simulink model "Slip_Ratio_Controller"  (R2018b)
settings: Solver=FixedStepAuto  StartTime=0.0  StopTime=10.0  FixedStep=global_time_step  RelTol=1e-3
undefined symbols (not defined in the file): Area, Cd, DiscIntNeverNeededParam, Jw, Mass, Q, r, R, rho, SRC_Ts, tyre_radius
libraries: simulink x2, peGeneralControl x1
settings Model: PauseTimes=1  Creator=univ4123  LastModifiedBy=univ4123
settings RTWCC: GenCodeOnly=on  Toolchain=MinGW64 | gmake (64-bit Windows)

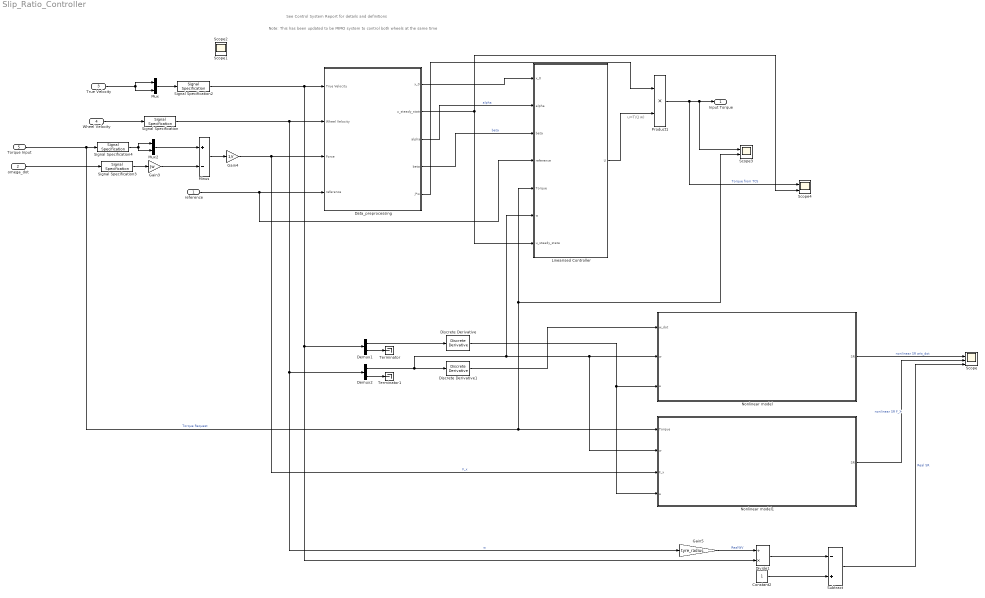
== system Slip_Ratio_Controller ==
  note: Note: This has been updated to be MIMO system to control both wheels at the same time
  note: See Control System Report for details and definitions
  note: u=T/(J w)
  reference : Inport
  omega_dot : Inport  Port=2
  True Velocity : Inport  Port=3
  Wheel Velocity : Inport  Port=4
  Torque Input : Inport  Port=5
  Constant2 : Constant  SampleTime=SRC_Ts
  Data_preprocessing : Subsystem
  Demux1 : Demux  Outputs=2
  Demux2 : Demux  Outputs=2
  Discrete Derivative : simulink/Discrete/Discrete Derivative  gainval=1.0  ICPrevScaledInput=0.0  OutMin=[]  OutMax=[]  OutDataType=fixdt(1, 16)  OutScaling=2^-10  DoSatur=off
  Discrete Derivative1 : simulink/Discrete/Discrete Derivative  gainval=1.0  ICPrevScaledInput=0.0  OutMin=[]  OutMax=[]  OutDataType=fixdt(1, 16)  OutScaling=2^-10  DoSatur=off
  Divide1 : Product  Inputs=/*
  Gain3 : Gain  Gain=Jw
  Gain4 : Gain  Gain=1/r
  Gain5 : Gain  Gain=tyre_radius
  Linearised Controller : Subsystem
  Minus : Sum  Inputs=+-
  Mux : Mux  Inputs=2
  Mux2 : Mux  Inputs=2
  Nonlinear model : Subsystem
  Nonlinear model1 : Subsystem
  Product1 : Product
  Scope : Scope  NumInputPorts=4
  Scope3 : Scope  NumInputPorts=2
  Scope4 : Scope  NumInputPorts=2
  Signal Specification : SignalSpecification  Dimensions=[2,1]
  Signal Specification2 : SignalSpecification  Dimensions=[2,1]
  Signal Specification3 : SignalSpecification  Dimensions=[2,1]
  Signal Specification4 : SignalSpecification  Dimensions=1
  Subtract : Sum  Inputs=-+
  Terminator : Terminator
  Terminator1 : Terminator
  Input Torque : Outport
  Scope1 : Scope
  Scope2 : Scope
  wires:
  Wheel Velocity/1 -> Signal Specification/1
  Data_preprocessing/2(u_steady_state) -> Scope4/2, Linearised Controller/7(u_steady_state)
  Linearised Controller/1(U) -> Product1/2
  Product1/1 -> Scope4/1, Scope3/1, Input Torque/1  "Torque from TCS"
  reference/1 -> Linearised Controller/4(reference), Data_preprocessing/4(reference)
  True Velocity/1 -> Mux/2, Mux/1
  Gain4/1 -> Nonlinear model1/3(F_x), Data_preprocessing/3(Force)  "F_x"
  Nonlinear model/1(SR) -> Scope/2  "nonlinear SR w/w_dot"
  Demux1/2 -> Terminator/1
  Demux2/2 -> Terminator1/1
  Torque Input/1 -> Nonlinear model1/1(Torque), Linearised Controller/5(Torque), Scope3/2, Signal Specification4/1  "Torque Request"
  Demux1/1 -> Discrete Derivative/1
  Demux2/1 -> Nonlinear model1/2(w), Nonlinear model/2(w), Linearised Controller/6(w), Discrete Derivative1/1
  Discrete Derivative/1 -> Nonlinear model1/4(a), Nonlinear model/3(a)
  Discrete Derivative1/1 -> Nonlinear model/1(w_dot)
  Gain3/1 -> Minus/2
  Minus/1 -> Gain4/1
  omega_dot/1 -> Signal Specification3/1
  Mux2/1 -> Minus/1
  Signal Specification3/1 -> Gain3/1
  Signal Specification4/1 -> Mux2/1, Mux2/2
  Nonlinear model1/1(SR) -> Scope/3  "nonlinear SR F_X"
  Signal Specification/1 -> Gain5/1, Demux2/1, Data_preprocessing/2(Wheel Velocity)  "w"
  Divide1/1 -> Subtract/1
  Mux/1 -> Signal Specification2/1
  Gain5/1 -> Divide1/1  "RealWV"
  Constant2/1 -> Subtract/2
  Subtract/1 -> Scope/4  "Real SR"
  Signal Specification2/1 -> Divide1/2, Demux1/1, Data_preprocessing/1(True Velocity)
  Data_preprocessing/1(x_0) -> Linearised Controller/1(x_0)
  Data_preprocessing/3(alpha) -> Linearised Controller/2(alpha)  "alpha"
  Data_preprocessing/4(beta) -> Linearised Controller/3(beta)  "beta"
  Data_preprocessing/5(J*w) -> Product1/1

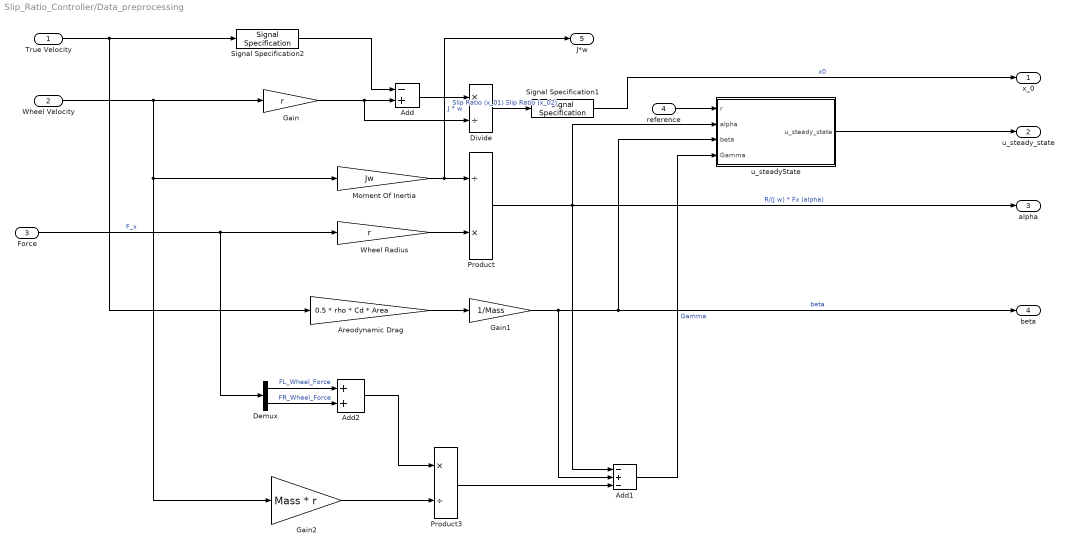
== system Slip_Ratio_Controller/Data_preprocessing ==
  True Velocity : Inport
  Wheel Velocity : Inport  Port=2
  Force : Inport  Port=3
  reference : Inport  Port=4
  Add : Sum  Inputs=-+
  Add1 : Sum  Inputs=-+-
  Add2 : Sum
  Areodynamic Drag : Gain  Gain=0.5 * rho * Cd * Area
  Demux : Demux  Outputs=2
  Divide : Product  Inputs=*/
  Gain : Gain  Gain=r
  Gain1 : Gain  Gain=1/Mass
  Gain2 : Gain  Gain=Mass * r
  Moment Of Inertia : Gain  Gain=Jw
  Product : Product  Inputs=/*
  Product3 : Product  Inputs=*/
  Signal Specification1 : SignalSpecification  Dimensions=[2,1]
  Signal Specification2 : SignalSpecification  Dimensions=[2,1]
  Wheel Radius : Gain  Gain=r
  u_steadyState : Subsystem
  x_0 : Outport
  u_steady_state : Outport  Port=2
  alpha : Outport  Port=3
  beta : Outport  Port=4
  J*w : Outport  Port=5
  wires:
  True Velocity/1 -> Signal Specification2/1, Areodynamic Drag/1
  Signal Specification2/1 -> Add/1
  Wheel Velocity/1 -> Gain/1, Moment Of Inertia/1, Gain2/1
  Product/1 -> u_steadyState/2(alpha), alpha/1, Add1/1  "R/(J w) * Fx (alpha)"
  Moment Of Inertia/1 -> J*w/1, Product/1  "J * w"
  Gain/1 -> Divide/2, Add/2
  Divide/1 -> Signal Specification1/1  "Slip Ratio (x_01) Slip Ratio (x_02)"
  Wheel Radius/1 -> Product/2
  Gain1/1 -> u_steadyState/3(beta), beta/1, Add1/2  "beta"
  Add1/1 -> u_steadyState/4(Gamma)  "Gamma"
  Demux/2 -> Add2/2  "FR_Wheel_Force"
  Add2/1 -> Product3/1
  Gain2/1 -> Product3/2
  Signal Specification1/1 -> x_0/1  "x0"
  Force/1 -> Demux/1, Wheel Radius/1  "F_x"
  Areodynamic Drag/1 -> Gain1/1
  Product3/1 -> Add1/3
  Demux/1 -> Add2/1  "FL_Wheel_Force"
  Add/1 -> Divide/1
  u_steadyState/1(u_steady_state) -> u_steady_state/1
  reference/1 -> u_steadyState/1(r)

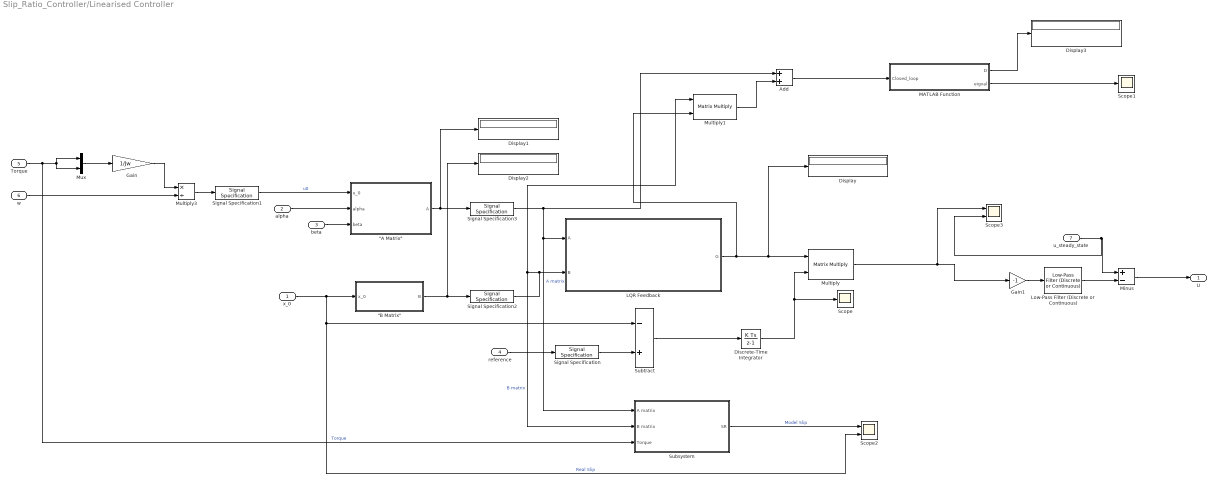
== system Slip_Ratio_Controller/Linearised Controller ==
  x_0 : Inport
  alpha : Inport  Port=2
  beta : Inport  Port=3
  reference : Inport  Port=4
  Torque : Inport  Port=5
  w : Inport  Port=6
  u_steady_state : Inport  Port=7
  "\"A Matrix\"" : Subsystem
  "\"B Matrix\"" : Subsystem
  Add : Sum
  Discrete-Time Integrator : DiscreteIntegrator  SampleTime=-1  ICPrevOutput=DiscIntNeverNeededParam  ICPrevScaledInput=DiscIntNeverNeededParam
  Display{,1..3} (4 alike) : Display
  Gain : Gain  Gain=1/Jw
  Gain1 : Gain  Gain=-1
  LQR Feedback : Subsystem
  Low-Pass Filter (Discrete or Continuous) : peGeneralControl/Low-Pass Filter (Discrete or Continuous)  K=1  T=10  B=inf  A=-inf  Ts=-1
  MATLAB Function : MATLAB Function  TreatAsAtomicUnit=on
  Minus : Sum  Inputs=+-
  Multiply : Product  Multiplication=Matrix(*)
  Multiply1 : Product  Multiplication=Matrix(*)
  Multiply3 : Product  Inputs=*/
  Mux : Mux  Inputs=2
  Scope : Scope
  Scope1 : Scope
  Scope2 : Scope  NumInputPorts=2
  Scope3 : Scope  NumInputPorts=2
  Signal Specification : SignalSpecification  Dimensions=[2 1]
  Signal Specification1 : SignalSpecification  Dimensions=[2,1]
  Signal Specification2 : SignalSpecification  Dimensions=[2,2]
  Signal Specification3 : SignalSpecification  Dimensions=[2,2]
  Subsystem : Subsystem
  Subtract : Sum  Inputs=-+
  U : Outport
  wires:
  alpha/1 -> "\"A Matrix\""/2(alpha)
  beta/1 -> "\"A Matrix\""/3(beta)
  x_0/1 -> Scope2/2, Subtract/1, "\"B Matrix\""/1(x_0)  "Real Slip"
  "\"A Matrix\""/1(A) -> Display1/1, Signal Specification3/1
  "\"B Matrix\""/1(B) -> Display2/1, Signal Specification2/1
  reference/1 -> Signal Specification/1
  Signal Specification2/1 -> LQR Feedback/2(B), Subsystem/2(B matrix), Multiply1/1  "B matrix"
  Signal Specification3/1 -> Add/1, Subsystem/1(A matrix), LQR Feedback/1(A)  "A matrix"
  Multiply3/1 -> Signal Specification1/1
  Gain/1 -> Multiply3/1
  w/1 -> Multiply3/2
  Torque/1 -> Subsystem/3(Torque), Mux/2, Mux/1  "Torque"
  Mux/1 -> Gain/1
  Signal Specification/1 -> Subtract/2
  Signal Specification1/1 -> "\"A Matrix\""/1(u_0)  "u0"
  Low-Pass Filter (Discrete or Continuous)/1 -> Minus/2
  Gain1/1 -> Low-Pass Filter (Discrete or Continuous)/1
  Multiply/1 -> Scope3/1, Gain1/1
  Minus/1 -> U/1
  Subtract/1 -> Discrete-Time Integrator/1
  Discrete-Time Integrator/1 -> Multiply/2, Scope/1
  LQR Feedback/1(G) -> Multiply1/2, Display/1, Multiply/1
  Multiply1/1 -> Add/2
  Add/1 -> MATLAB Function/1(Closed_loop)
  MATLAB Function/1(D) -> Display3/1
  MATLAB Function/2(eigval) -> Scope1/1
  Subsystem/1(SR) -> Scope2/1  "Model Slip"
  u_steady_state/1 -> Scope3/2, Minus/1

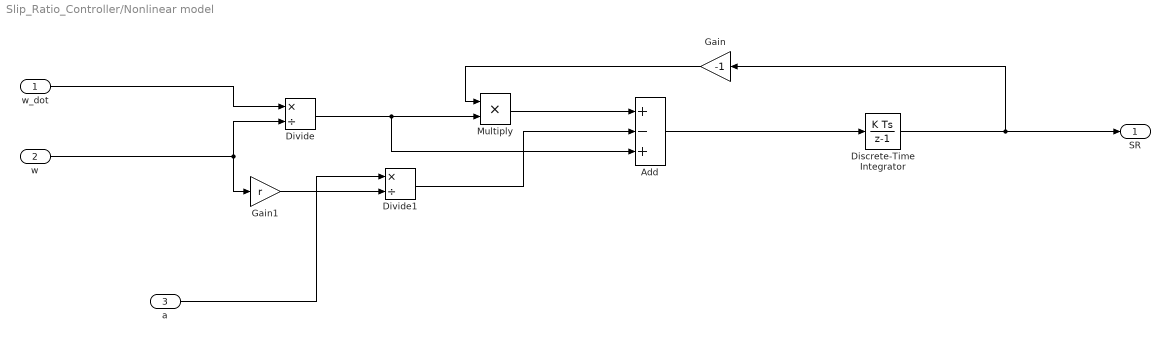
== system Slip_Ratio_Controller/Nonlinear model ==
  w_dot : Inport
  w : Inport  Port=2
  a : Inport  Port=3
  Add : Sum  Inputs=+-+
  Discrete-Time Integrator : DiscreteIntegrator  SampleTime=-1  ICPrevOutput=DiscIntNeverNeededParam  ICPrevScaledInput=DiscIntNeverNeededParam
  Divide : Product  Inputs=*/
  Divide1 : Product  Inputs=*/
  Gain : Gain  Gain=-1
  Gain1 : Gain  Gain=r
  Multiply : Product
  SR : Outport
  wires:
  w_dot/1 -> Divide/1
  w/1 -> Divide/2, Gain1/1
  Gain1/1 -> Divide1/2
  Divide/1 -> Add/3, Multiply/2
  Gain/1 -> Multiply/1
  Multiply/1 -> Add/1
  a/1 -> Divide1/1
  Divide1/1 -> Add/2
  Add/1 -> Discrete-Time Integrator/1
  Discrete-Time Integrator/1 -> Gain/1, SR/1

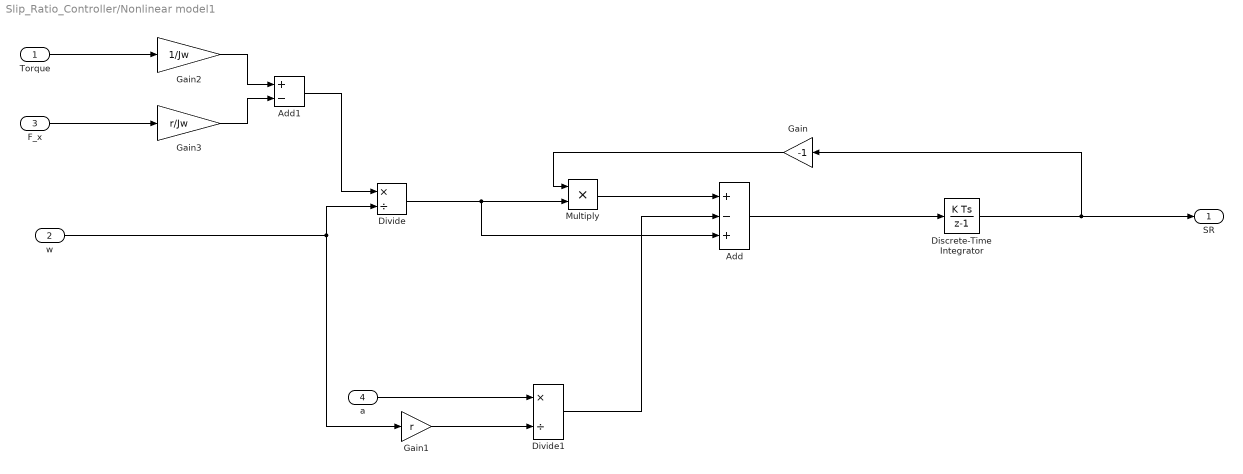
== system Slip_Ratio_Controller/Nonlinear model1 ==
  Torque : Inport
  w : Inport  Port=2
  F_x : Inport  Port=3
  a : Inport  Port=4
  Add : Sum  Inputs=+-+
  Add1 : Sum  Inputs=+-
  Discrete-Time Integrator : DiscreteIntegrator  SampleTime=-1  ICPrevOutput=DiscIntNeverNeededParam  ICPrevScaledInput=DiscIntNeverNeededParam
  Divide : Product  Inputs=*/
  Divide1 : Product  Inputs=*/
  Gain : Gain  Gain=-1
  Gain1 : Gain  Gain=r
  Gain2 : Gain  Gain=1/Jw
  Gain3 : Gain  Gain=r/Jw
  Multiply : Product
  SR : Outport
  wires:
  Torque/1 -> Gain2/1
  w/1 -> Gain1/1, Divide/2
  Gain1/1 -> Divide1/2
  Divide/1 -> Add/3, Multiply/2
  Gain/1 -> Multiply/1
  Multiply/1 -> Add/1
  a/1 -> Divide1/1
  Divide1/1 -> Add/2
  Add/1 -> Discrete-Time Integrator/1
  Discrete-Time Integrator/1 -> Gain/1, SR/1
  F_x/1 -> Gain3/1
  Gain2/1 -> Add1/1
  Gain3/1 -> Add1/2
  Add1/1 -> Divide/1

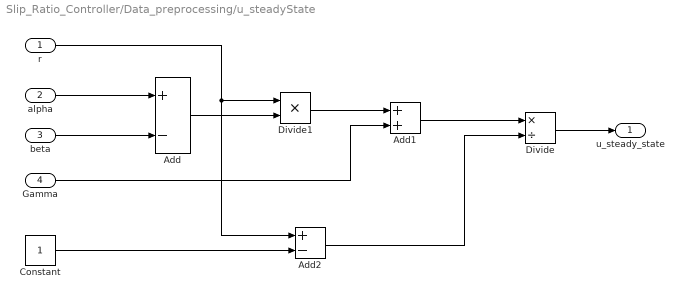
== system Slip_Ratio_Controller/Data_preprocessing/u_steadyState ==
  r : Inport
  alpha : Inport  Port=2
  beta : Inport  Port=3
  Gamma : Inport  Port=4
  Add : Sum  Inputs=+-
  Add1 : Sum
  Add2 : Sum  Inputs=+-
  Constant : Constant  SampleTime=SRC_Ts
  Divide : Product  Inputs=*/
  Divide1 : Product  Inputs=**
  u_steady_state : Outport
  wires:
  Divide/1 -> u_steady_state/1
  Add/1 -> Divide1/2
  alpha/1 -> Add/1
  beta/1 -> Add/2
  r/1 -> Add2/1, Divide1/1
  Divide1/1 -> Add1/1
  Gamma/1 -> Add1/2
  Add1/1 -> Divide/1
  Constant/1 -> Add2/2
  Add2/1 -> Divide/2

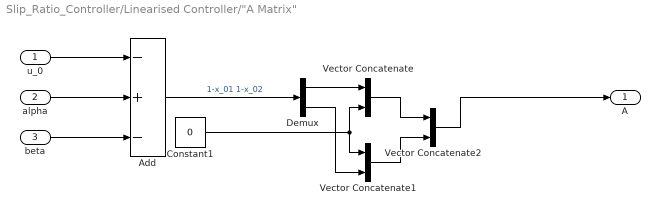
== system Slip_Ratio_Controller/Linearised Controller/"A Matrix" ==
  u_0 : Inport
  alpha : Inport  Port=2
  beta : Inport  Port=3
  Add : Sum  Inputs=-+-
  Constant1 : Constant  Value=0  SampleTime=SRC_Ts
  Demux : Demux  Outputs=2
  Vector Concatenate : Concatenate  ConcatenateDimension=2
  Vector Concatenate1 : Concatenate
  Vector Concatenate2 : Concatenate  Mode=Multidimensional array  ConcatenateDimension=2
  A : Outport
  wires:
  u_0/1 -> Add/1
  alpha/1 -> Add/2
  beta/1 -> Add/3
  Demux/2 -> Vector Concatenate1/2
  Add/1 -> Demux/1  "1-x_01 1-x_02"
  Constant1/1 -> Vector Concatenate1/1, Vector Concatenate/2
  Vector Concatenate1/1 -> Vector Concatenate2/2
  Vector Concatenate2/1 -> A/1
  Demux/1 -> Vector Concatenate/1
  Vector Concatenate/1 -> Vector Concatenate2/1

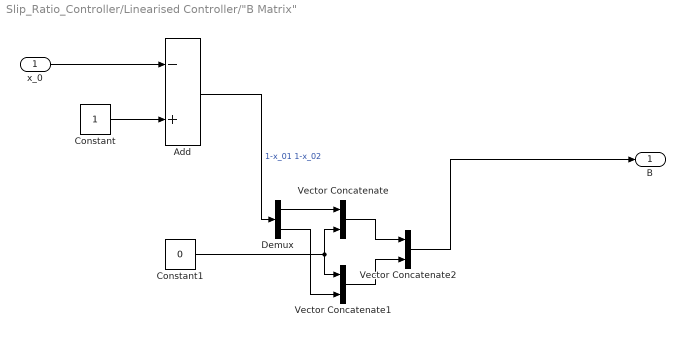
== system Slip_Ratio_Controller/Linearised Controller/"B Matrix" ==
  x_0 : Inport
  Add : Sum  Inputs=-+
  Constant : Constant  SampleTime=SRC_Ts
  Constant1 : Constant  Value=0  SampleTime=SRC_Ts
  Demux : Demux  Outputs=2
  Vector Concatenate : Concatenate  ConcatenateDimension=2
  Vector Concatenate1 : Concatenate
  Vector Concatenate2 : Concatenate  Mode=Multidimensional array  ConcatenateDimension=2
  B : Outport
  wires:
  Constant/1 -> Add/2
  Add/1 -> Demux/1  "1-x_01 1-x_02"
  Demux/1 -> Vector Concatenate/1
  Demux/2 -> Vector Concatenate1/2
  Constant1/1 -> Vector Concatenate1/1, Vector Concatenate/2
  Vector Concatenate1/1 -> Vector Concatenate2/2
  Vector Concatenate/1 -> Vector Concatenate2/1
  Vector Concatenate2/1 -> B/1
  x_0/1 -> Add/1

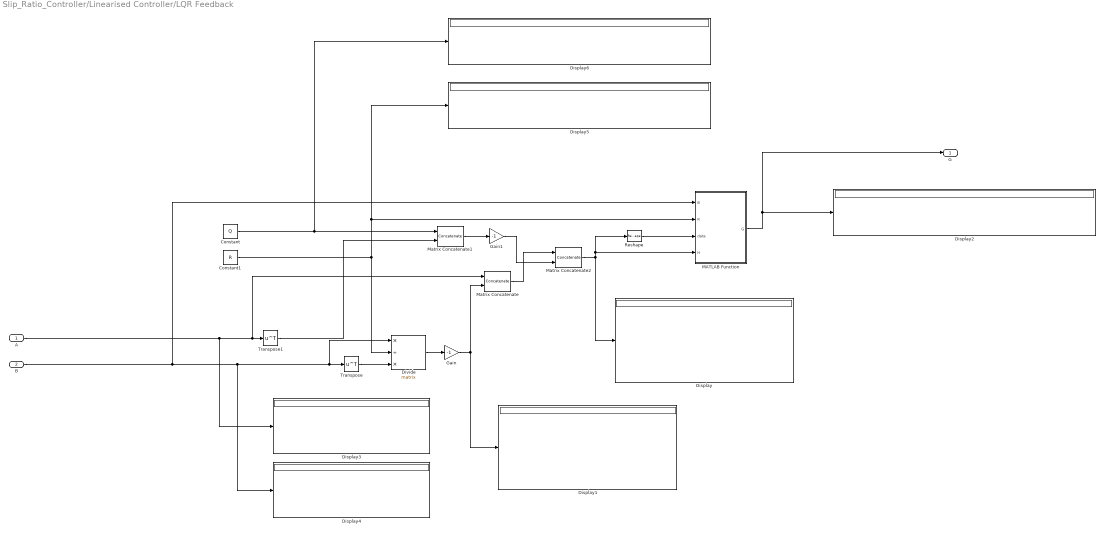
== system Slip_Ratio_Controller/Linearised Controller/LQR Feedback ==
  A : Inport
  B : Inport  Port=2
  Constant : Constant  Value=Q  SampleTime=SRC_Ts
  Constant1 : Constant  Value=R  SampleTime=SRC_Ts
  Display{,1..6} (7 alike) : Display
  Divide : Product  Inputs=*/*  Multiplication=Matrix(*)
  Gain : Gain  Gain=-1
  Gain1 : Gain  Gain=-1
  MATLAB Function : MATLAB Function  TreatAsAtomicUnit=on
  Matrix Concatenate : Concatenate  Mode=Multidimensional array  ConcatenateDimension=2
  Matrix Concatenate1 : Concatenate  Mode=Multidimensional array  ConcatenateDimension=2
  Matrix Concatenate2 : Concatenate  Mode=Multidimensional array
  Reshape : Reshape
  Transpose : Math  Operator=transpose  SaturateOnIntegerOverflow=on
  Transpose1 : Math  Operator=transpose  SaturateOnIntegerOverflow=on
  G : Outport
  wires:
  B/1 -> Display4/1, Divide/1, Transpose/1, MATLAB Function/1(B)
  Constant1/1 -> Divide/2, Display5/1, MATLAB Function/2(R)
  Transpose/1 -> Divide/3
  Constant/1 -> Display6/1, Matrix Concatenate1/1
  A/1 -> Display3/1, Matrix Concatenate/1, Transpose1/1
  Transpose1/1 -> Matrix Concatenate1/2
  Divide/1 -> Gain/1
  Gain/1 -> Matrix Concatenate/2, Display1/1
  Matrix Concatenate1/1 -> Gain1/1
  Gain1/1 -> Matrix Concatenate2/2
  Matrix Concatenate/1 -> Matrix Concatenate2/1
  Matrix Concatenate2/1 -> Reshape/1, MATLAB Function/4(H), Display/1
  MATLAB Function/1(G) -> G/1, Display2/1
  Reshape/1 -> MATLAB Function/3(data)

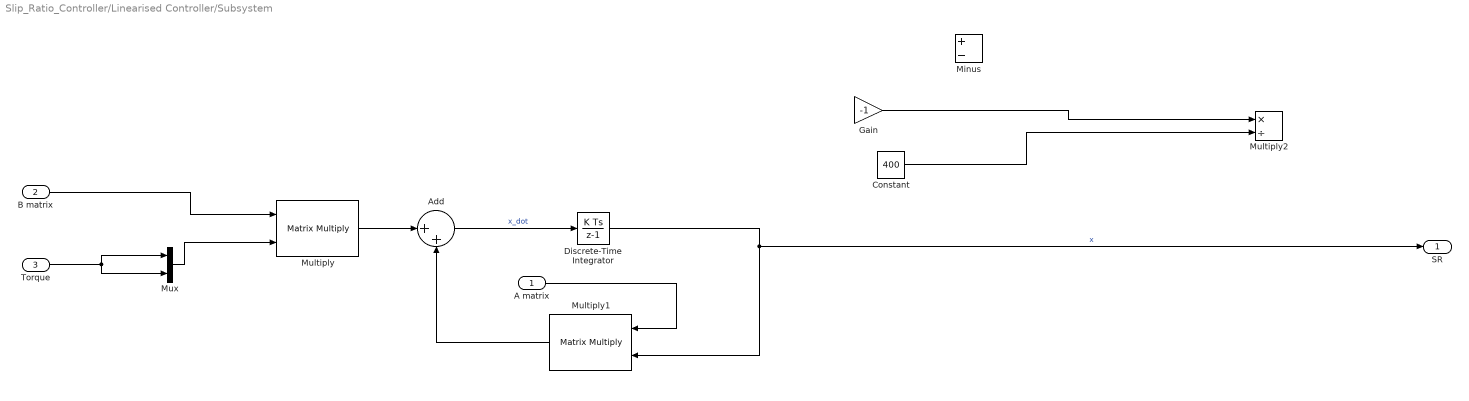
== system Slip_Ratio_Controller/Linearised Controller/Subsystem ==
  A matrix : Inport
  B matrix : Inport  Port=2
  Torque : Inport  Port=3
  Add : Sum  Inputs=|++
  Constant : Constant  Value=400
  Discrete-Time Integrator : DiscreteIntegrator  SampleTime=SRC_Ts  ICPrevOutput=DiscIntNeverNeededParam  ICPrevScaledInput=DiscIntNeverNeededParam
  Gain : Gain  Gain=-1
  Minus : Sum  Inputs=+-
  Multiply : Product  Multiplication=Matrix(*)
  Multiply1 : Product  Multiplication=Matrix(*)
  Multiply2 : Product  Inputs=*/
  Mux : Mux  Inputs=2
  SR : Outport
  wires:
  B matrix/1 -> Multiply/1
  Mux/1 -> Multiply/2
  A matrix/1 -> Multiply1/1
  Multiply1/1 -> Add/2
  Multiply/1 -> Add/1
  Add/1 -> Discrete-Time Integrator/1  "x_dot"
  Discrete-Time Integrator/1 -> SR/1, Multiply1/2  "x"
  Torque/1 -> Mux/2, Mux/1
  Constant/1 -> Multiply2/2
  Gain/1 -> Multiply2/1

== matlab function Slip_Ratio_Controller/Linearised Controller/LQR Feedback/MATLAB Function ==
  data: B input; R input; data input; H input; G output
function G = LQR(B, R, data, H)
if any(isnan(data))
    G=[0 0; 0 0];
elseif any(data == Inf)
    G=[0 0; 0 0];
else
    [V,D] = eig(H);
    
    stable = D(:,:) < 0;
    
    [~, col] = find(stable);
    
    W_1 = V(:,col(1));
    W_2 = V(:,col(2));
    W_ = [W_1 W_2];
    
    W11 = W_(1:2,:);
    W12 = W_(3:4,:);
    
    P = W12/W11;
    
    G = inv(R)* B' * real(P);
    
end

== matlab function Slip_Ratio_Controller/Linearised Controller/MATLAB Function ==
  data: Closed_loop input; D output; eigval output
function [D,eigval] = fcn(Closed_loop)

[~,D] = eig(Closed_loop);

eigval = real(D(1,1));
